simulink model "EffLookup45kWEMotor"  (Simulink 7.7)
settings: Solver=ode45  StartTime=0.0  StopTime=10.0  RelTol=1e-3
settings Model: Creator=Arjun  LastModifiedBy=Arjun

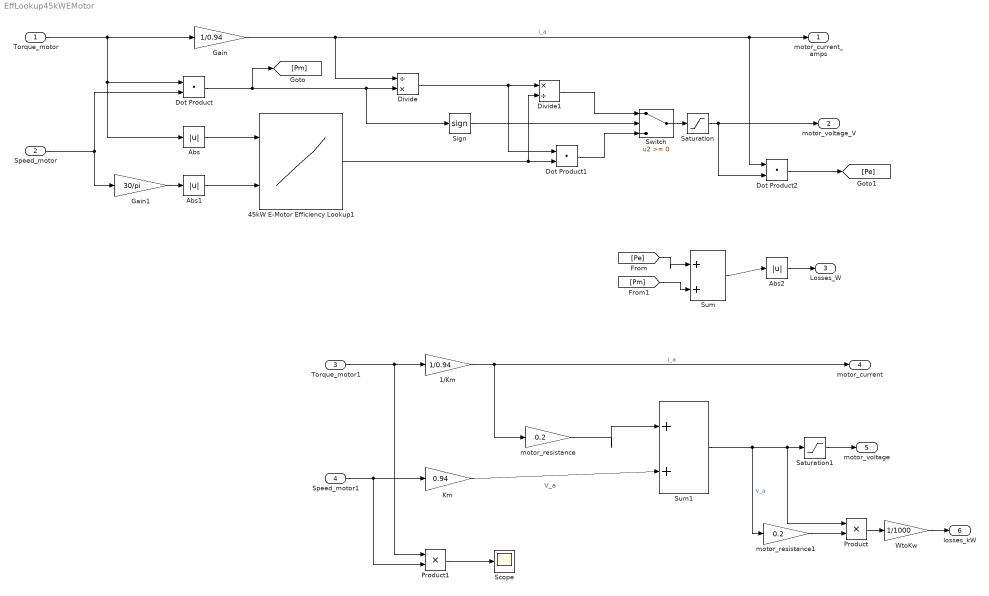
== system EffLookup45kWEMotor ==
  note: V_a
  Torque_motor : Inport
  Speed_motor : Inport  Port=2
  Torque_motor1 : Inport  Port=3
  Speed_motor1 : Inport  Port=4
  1/Km : Gain  Gain=1/0.94
  45kW E-Motor Efficiency Lookup1 : Lookup2D  RowIndex=[0,50,100,150,200,250,300,350,400,400,500,550]  ColumnIndex=[0,500,1000,1500,2000,2050,3000,3500,4000,4500]  Table=reshape([0.5,0.7,0.73,0.72,0.72,0.69,0.68,0.67,0.62,0.6,0.55,0.5,0.5,0.7,0.81,0.82,0.82,0.82,0.81,0.8,0.78,0.78,0.76,0.75,0.5,0.78,0.85,0.865,0.88,0.88,0.865,0.875,0.87,0.86,0.855,0.85,0.5,0.73,0.865,0.88,0.9,0.9,0.905,0.905,0.9,0.89,0.895,0.88,0.5,0.7,0.875,0.905,0.91,0.91,0.915,0.915,0.92,0.925,.925,0,0.5,0.8,0.875,0.905,0.915,0.92,0.92,0.925,0.93,0.93,0,0,0.5,0.76,0.875,0.9,0.925,0.94,0.95,0.96,0,0,0,0,0.5,0.76,0.875,0.9,0.925,0.935,0.935,0,0,0,0,0,0.5,0.75,0.87,0.905,0.925,0.925,0,0,0,0,0,0,0.5,0.75,0.865,0.905,0.92,0.92,0,0,0,0,0,0],12,10)
  Abs : Abs
  Abs1 : Abs
  Abs2 : Abs
  Divide : Product  Inputs=/*
  Divide1 : Product  Inputs=*/
  Dot Product : DotProduct  InputSameDT=on  OutDataTypeStr=Inherit: Inherit via internal rule
  Dot Product1 : DotProduct  InputSameDT=on  OutDataTypeStr=Inherit: Inherit via internal rule
  Dot Product2 : DotProduct  InputSameDT=on  OutDataTypeStr=Inherit: Inherit via internal rule
  Gain : Gain  Gain=1/0.94
  Gain1 : Gain  Gain=30/pi
  Km : Gain  Gain=0.94
  Product : Product  RndMeth=Zero
  Product1 : Product  RndMeth=Zero
  Saturation : Saturate  UpperLimit=300  LowerLimit=0
  Saturation1 : Saturate  UpperLimit=300  LowerLimit=0
  Scope : Scope
  Sign : Signum
  Sum : Sum  Inputs=|++
  Sum1 : Sum  Inputs=|++
  Switch : Switch
  WtoKw : Gain  Gain=1/1000
  motor_resistance : Gain  Gain=0.2
  motor_resistance1 : Gain  Gain=0.2
  motor_current_amps : Outport
  motor_voltage_V : Outport  Port=2
  Losses_W : Outport  Port=3
  motor_current : Outport  Port=4
  motor_voltage : Outport  Port=5
  losses_kW : Outport  Port=6
  wires:
  Torque_motor/1 -> Gain/1, Abs/1, Dot Product/1
  Gain/1 -> Divide/1, motor_current_amps/1, Dot Product2/1  "i_a"
  Abs/1 -> 45kW E-Motor Efficiency Lookup1/1
  Abs1/1 -> 45kW E-Motor Efficiency Lookup1/2
  Speed_motor/1 -> Dot Product/2, Gain1/1
  Dot Product/1 -> Divide/2, Sign/1, [Pm]
  Divide/1 -> Divide1/1, Dot Product1/1
  45kW E-Motor Efficiency Lookup1/1 -> Dot Product1/2, Divide1/2
  Sign/1 -> Switch/2
  Divide1/1 -> Switch/1
  Dot Product1/1 -> Switch/3
  Switch/1 -> Saturation/1
  Dot Product2/1 -> [Pe]
  [Pe] -> Sum/1
  [Pm] -> Sum/2
  Sum/1 -> Abs2/1
  Abs2/1 -> Losses_W/1
  Gain1/1 -> Abs1/1
  Saturation/1 -> motor_voltage_V/1, Dot Product2/2
  Torque_motor1/1 -> 1/Km/1, Product1/1
  Speed_motor1/1 -> Km/1, Product1/2
  Km/1 -> Sum1/2
  1/Km/1 -> motor_resistance/1, motor_current/1  "i_a"
  motor_resistance/1 -> Sum1/1
  Sum1/1 -> motor_resistance1/1, Product/1, Saturation1/1  "v_a"
  motor_resistance1/1 -> Product/2
  Product/1 -> WtoKw/1
  WtoKw/1 -> losses_kW/1
  Saturation1/1 -> motor_voltage/1
  Product1/1 -> Scope/1
